simulink model "complete_controller"  (R2023a)
settings: Solver=FixedStepAuto  StartTime=0.0  StopTime=inf  FixedStep=0.01  RelTol=1e-3
model workspace (MAT data in the model file):
  SL_ROS_VariableLengthArrays_MaxSizes : object (value not decoded)
undefined symbols (not defined in the file): Btrigger_boost, DAapply_nudges, DAdesired_pose, DAff_body_force, DAsolver_weights, Djoy_R_X, Dreverse_throttle, Dthrottle, Iangular_mode, Ilinear_mode
libraries: ros2lib x76, utils x1, mpclib x1
(part 2 of 2)

== matlab function complete_controller/Subsystem/RPM Conversion ==
  data: requestedForces input; RPMs output; coefficents input; tableMode input
function RPMs = fcn(requestedForces, coefficents, tableMode)

%coefficents come from param bus

%the output array with rpm values
RPMs = zeros([8,1]);

if(tableMode)
   %evaluate each thruster -- discontinuos curve
    for i = 1:8
        requestedForce = requestedForces(i);
        RPMs(i) = ((-500 * exp((-1/2) * abs(requestedForce))) + 500) * sign(requestedForce);
    end 

else

    %evaluate each thruster -- discontinuos curve
    for i = 1:8
        requestedForce = requestedForces(i);
        
        if(requestedForce > 0)
            %positive curve
            RPMs(i) = round(coefficents(1) + coefficents(2) * requestedForces(i) + coefficents(3) * tanh(requestedForces(i)) + requestedForces(i)^(1/4) * coefficents(4));
        else
            %negative curve
            RPMs(i) = round(coefficents(5) + coefficents(6) * requestedForces(i) + coefficents(7) * tanh(requestedForces(i)) + abs(requestedForces(i))^(1/4) * coefficents(8));
        end
    
    end

end
